simulink model "sysF_LA"  (R2023a)
settings: Solver=ode15s  StartTime=0.0  StopTime=20  MaxStep=1e-3  RelTol=1e-3  AbsTol=1e-5
settings Model: Creator=miros  LastModifiedBy=miros
settings DataIOCC: ReturnWorkspaceOutputs=off
settings DebuggingCC: AlgebraicLoopMsg=none  ArtificialAlgebraicLoopMsg=none  BlockPriorityViolationMsg=error  MinStepSizeMsg=error  MaxConsecutiveZCsMsg=none  ModelReferenceExtraNoncontSigs=none  OperatingPointInterfaceChecksumMismatchMsg=none

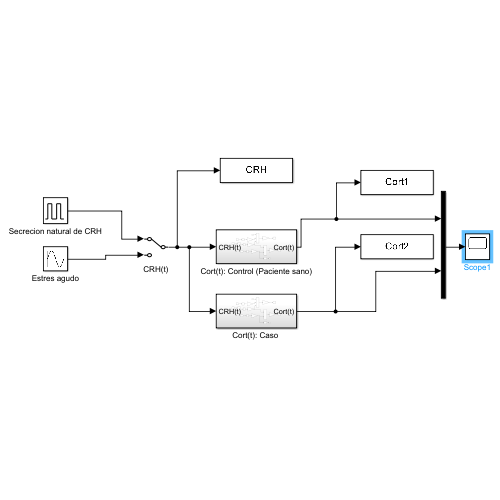
[thumbnail: Simulink's stored preview of the top-level diagram]
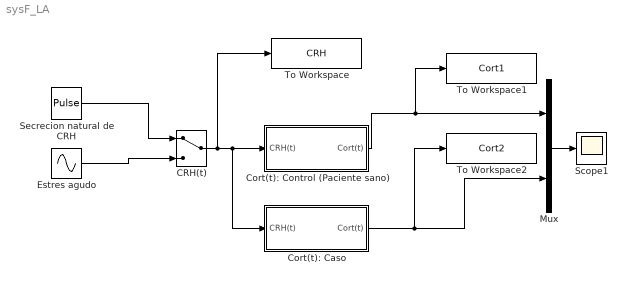
== system sysF_LA ==
  CRH(t) : ManualSwitch
  "Cort(t): Caso " : Subsystem
  Cort(t): Control (Paciente sano) : Subsystem
  Estres agudo : Sin  Amplitude=2.5  Frequency=pi  SampleTime=0
  Mux : Mux  Inputs=2
  Scope1 : Scope
  Secrecion natural de CRH : DiscretePulseGenerator  PulseType=Time based  Amplitude=4  Period=1/0.5  PulseWidth=50  PhaseDelay=1
  To Workspace : ToWorkspace  VariableName=CRH  SampleTime=-1
  To Workspace1 : ToWorkspace  VariableName=Cort1  SampleTime=-1
  To Workspace2 : ToWorkspace  VariableName=Cort2  SampleTime=-1
  wires:
  Secrecion natural de CRH/1 -> CRH(t)/1
  Estres agudo/1 -> CRH(t)/2
  CRH(t)/1 -> To Workspace/1, "Cort(t): Caso "/1(CRH(t)), Cort(t): Control (Paciente sano)/1(CRH(t))
  Mux/1 -> Scope1/1
  Cort(t): Control (Paciente sano)/1(Cort(t)) -> To Workspace1/1, Mux/1
  "Cort(t): Caso "/1(Cort(t)) -> To Workspace2/1, Mux/2

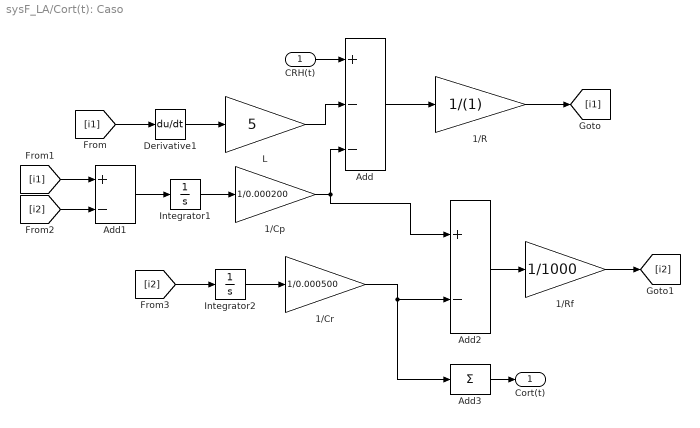
== system sysF_LA/Cort(t): Caso  ==
  CRH(t) : Inport
  1/Cp : Gain  Gain=1/0.000200
  1/Cr : Gain  Gain=1/0.000500
  1/R : Gain  Gain=1/(1)
  1/Rf : Gain  Gain=1/1000
  Add : Sum  Inputs=+--
  Add1 : Sum  Inputs=+-
  Add2 : Sum  Inputs=+-
  Add3 : Sum  Inputs=+
  Derivative1 : Derivative
  Integrator1 : Integrator
  Integrator2 : Integrator
  L : Gain  Gain=5
  Cort(t) : Outport
  wires:
  [i2] -> Integrator2/1
  Integrator2/1 -> 1/Cr/1
  Add1/1 -> Integrator1/1
  [i1] -> Derivative1/1
  Derivative1/1 -> L/1
  [i1] -> Add1/1
  1/Cp/1 -> Add2/1, Add/3
  Add2/1 -> 1/Rf/1
  1/Cr/1 -> Add2/2, Add3/1
  Add/1 -> 1/R/1
  L/1 -> Add/2
  [i2] -> Add1/2
  1/R/1 -> [i1]
  Integrator1/1 -> 1/Cp/1
  1/Rf/1 -> [i2]
  CRH(t)/1 -> Add/1
  Add3/1 -> Cort(t)/1

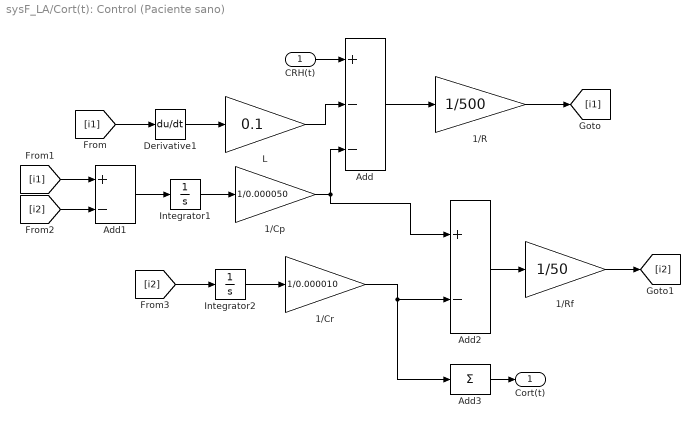
== system sysF_LA/Cort(t): Control (Paciente sano) ==
  CRH(t) : Inport
  1/Cp : Gain  Gain=1/0.000050
  1/Cr : Gain  Gain=1/0.000010
  1/R : Gain  Gain=1/500
  1/Rf : Gain  Gain=1/50
  Add : Sum  Inputs=+--
  Add1 : Sum  Inputs=+-
  Add2 : Sum  Inputs=+-
  Add3 : Sum  Inputs=+
  Derivative1 : Derivative
  Integrator1 : Integrator
  Integrator2 : Integrator
  L : Gain  Gain=0.1
  Cort(t) : Outport
  wires:
  [i2] -> Integrator2/1
  Integrator2/1 -> 1/Cr/1
  Add1/1 -> Integrator1/1
  [i1] -> Derivative1/1
  Derivative1/1 -> L/1
  [i1] -> Add1/1
  1/Cp/1 -> Add2/1, Add/3
  Add2/1 -> 1/Rf/1
  1/Cr/1 -> Add2/2, Add3/1
  Add/1 -> 1/R/1
  L/1 -> Add/2
  [i2] -> Add1/2
  1/R/1 -> [i1]
  Integrator1/1 -> 1/Cp/1
  1/Rf/1 -> [i2]
  CRH(t)/1 -> Add/1
  Add3/1 -> Cort(t)/1
